simulink model "GT_cruise"  (R2024a)
settings: Solver=ode4  StartTime=0.0  StopTime=10  FixedStep=1/1600  RelTol=1e-3
undefined symbols (not defined in the file): wind_x, wind_y, wind_z
libraries: GT x1, aerolibasang x1
settings Model: Creator=igmso  LastModifiedBy=igmso
settings DataIOCC: ExternalInput=[t,u]  InitialState=getstatestruct(op_trim3)  SaveFormat=StructureWithTime

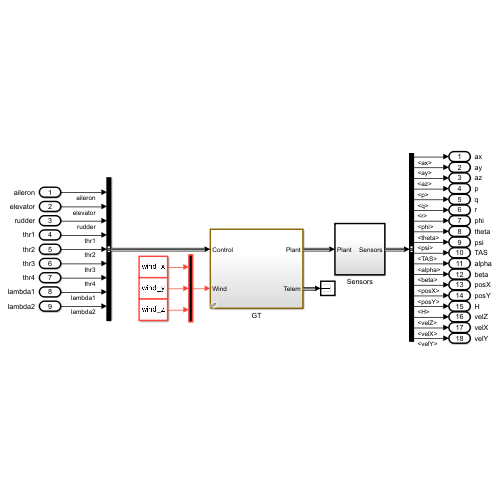
[thumbnail: Simulink's stored preview of the top-level diagram]
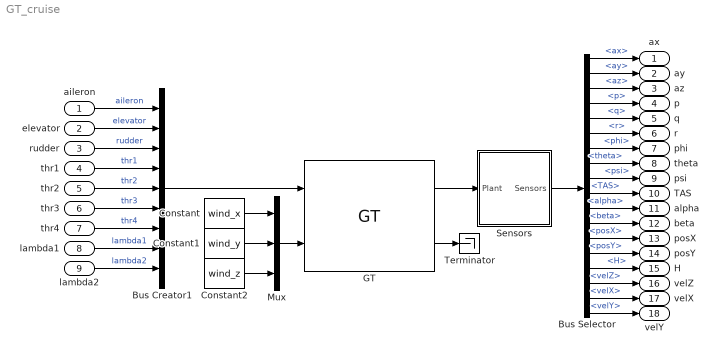
== system GT_cruise ==
  aileron : Inport
  elevator : Inport  Port=2
  rudder : Inport  Port=3
  thr1 : Inport  Port=4
  thr2 : Inport  Port=5
  thr3 : Inport  Port=6
  thr4 : Inport  Port=7
  lambda1 : Inport  Port=8
  lambda2 : Inport  Port=9
  Bus Creator1 : BusCreator  Inputs=9
  Bus Selector : BusSelector  OutputSignals=ax,ay,az,p,q,r,phi,theta,psi,TAS,alpha,beta,posX,posY,H,velZ,velX,velY
  Constant : Constant  Value=wind_x  SampleTime=-1
  Constant1 : Constant  Value=wind_y  SampleTime=-1
  Constant2 : Constant  Value=wind_z  SampleTime=-1
  GT : GT/GT  SystemSampleTime=-1  VariantActivationTime=update diagram  AllowFlexibleInterface=on  Latency=0  AutoFrameSizeCalculation=off
  Mux : Mux  Inputs=3
  Sensors : Subsystem
  Terminator : Terminator
  ax : Outport
  ay : Outport  Port=2
  az : Outport  Port=3
  p : Outport  Port=4
  q : Outport  Port=5
  r : Outport  Port=6
  phi : Outport  Port=7
  theta : Outport  Port=8
  psi : Outport  Port=9
  TAS : Outport  Port=10
  alpha : Outport  Port=11
  beta : Outport  Port=12
  posX : Outport  Port=13
  posY : Outport  Port=14
  H : Outport  Port=15
  velZ : Outport  Port=16
  velX : Outport  Port=17
  velY : Outport  Port=18
  wires:
  Bus Creator1/1 -> GT/1
  lambda2/1 -> Bus Creator1/9  "lambda2"
  lambda1/1 -> Bus Creator1/8  "lambda1"
  thr2/1 -> Bus Creator1/5  "thr2"
  thr3/1 -> Bus Creator1/6  "thr3"
  rudder/1 -> Bus Creator1/3  "rudder"
  thr1/1 -> Bus Creator1/4  "thr1"
  elevator/1 -> Bus Creator1/2  "elevator"
  aileron/1 -> Bus Creator1/1  "aileron"
  thr4/1 -> Bus Creator1/7  "thr4"
  Mux/1 -> GT/2
  Constant/1 -> Mux/1
  Constant1/1 -> Mux/2
  Constant2/1 -> Mux/3
  GT/2 -> Terminator/1
  GT/1 -> Sensors/1(Plant)
  Sensors/1(Sensors) -> Bus Selector/1
  Bus Selector/18 -> velY/1  "<velY>"
  Bus Selector/8 -> theta/1  "<theta>"
  Bus Selector/10 -> TAS/1  "<TAS>"
  Bus Selector/6 -> r/1  "<r>"
  Bus Selector/1 -> ax/1  "<ax>"
  Bus Selector/5 -> q/1  "<q>"
  Bus Selector/7 -> phi/1  "<phi>"
  Bus Selector/3 -> az/1  "<az>"
  Bus Selector/4 -> p/1  "<p>"
  Bus Selector/9 -> psi/1  "<psi>"
  Bus Selector/15 -> H/1  "<H>"
  Bus Selector/17 -> velX/1  "<velX>"
  Bus Selector/12 -> beta/1  "<beta>"
  Bus Selector/11 -> alpha/1  "<alpha>"
  Bus Selector/16 -> velZ/1  "<velZ>"
  Bus Selector/2 -> ay/1  "<ay>"
  Bus Selector/14 -> posY/1  "<posY>"
  Bus Selector/13 -> posX/1  "<posX>"

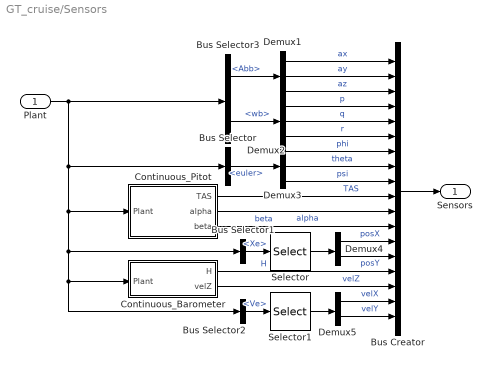
== system GT_cruise/Sensors ==
  Plant : Inport
  Bus Selector : BusSelector  OutputSignals=euler
  Bus Selector1 : BusSelector  OutputSignals=Xe
  Bus Selector2 : BusSelector  OutputSignals=Ve
  Bus Selector3 : BusSelector  OutputSignals=Abb,wb
  Bus Creator : BusCreator  Inputs=18
  Continuous_Barometer : Subsystem
  Continuous_Pitot : Subsystem
  Demux1 : Demux  Outputs=3
  Demux2 : Demux  Outputs=3
  Demux3 : Demux  Outputs=3
  Demux4 : Demux  Outputs=2
  Demux5 : Demux  Outputs=2
  Selector : Selector  InputPortWidth=3  IndexOptions=Index vector (dialog)  Indices=[1 2]  OutputSizes=1
  Selector1 : Selector  InputPortWidth=3  IndexOptions=Index vector (dialog)  Indices=[1 2]  OutputSizes=1
  Sensors : Outport
  wires:
  Continuous_Barometer/1(H) -> Bus Creator/15  "H"
  Continuous_Pitot/1(TAS) -> Bus Creator/10  "TAS"
  Continuous_Pitot/2(alpha) -> Bus Creator/11  "alpha"
  Continuous_Pitot/3(beta) -> Bus Creator/12  "beta"
  Demux1/3 -> Bus Creator/3  "az"
  Demux1/2 -> Bus Creator/2  "ay"
  Demux1/1 -> Bus Creator/1  "ax"
  Bus Selector3/1 -> Demux1/1  "<Abb>"
  Bus Selector3/2 -> Demux2/1  "<wb>"
  Demux2/1 -> Bus Creator/4  "p"
  Demux2/2 -> Bus Creator/5  "q"
  Demux2/3 -> Bus Creator/6  "r"
  Continuous_Barometer/2(velZ) -> Bus Creator/16  "velZ"
  Bus Selector/1 -> Demux3/1  "<euler>"
  Demux3/1 -> Bus Creator/7  "phi"
  Demux3/2 -> Bus Creator/8  "theta"
  Demux3/3 -> Bus Creator/9  "psi"
  Bus Selector1/1 -> Selector/1  "<Xe>"
  Selector/1 -> Demux4/1
  Demux4/1 -> Bus Creator/13  "posX"
  Demux4/2 -> Bus Creator/14  "posY"
  Bus Creator/1 -> Sensors/1
  Selector1/1 -> Demux5/1
  Bus Selector2/1 -> Selector1/1  "<Ve>"
  Plant/1 -> Bus Selector2/1, Continuous_Barometer/1(Plant), Bus Selector1/1, Continuous_Pitot/1(Plant), Bus Selector/1, Bus Selector3/1
  Demux5/1 -> Bus Creator/17  "velX"
  Demux5/2 -> Bus Creator/18  "velY"

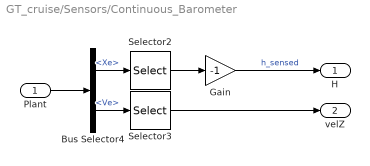
== system GT_cruise/Sensors/Continuous_Barometer ==
  Plant : Inport
  Bus Selector4 : BusSelector  OutputSignals=Xe,Ve
  Gain : Gain  Gain=-1
  Selector2 : Selector  InputPortWidth=3  IndexOptions=Index vector (dialog)  Indices=3  OutputSizes=1
  Selector3 : Selector  InputPortWidth=3  IndexOptions=Index vector (dialog)  Indices=3  OutputSizes=1
  H : Outport
  velZ : Outport  Port=2
  wires:
  Bus Selector4/1 -> Selector2/1  "<Xe>"
  Selector3/1 -> velZ/1
  Selector2/1 -> Gain/1
  Bus Selector4/2 -> Selector3/1  "<Ve>"
  Gain/1 -> H/1  "h_sensed"
  Plant/1 -> Bus Selector4/1

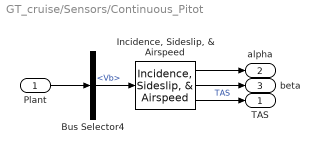
== system GT_cruise/Sensors/Continuous_Pitot ==
  Plant : Inport
  Bus Selector4 : BusSelector  OutputSignals=Vb
  "Incidence, Sideslip, & Airspeed" : aerolibasang/Incidence, Sideslip, & Airspeed
  TAS : Outport
  alpha : Outport  Port=2
  beta : Outport  Port=3
  wires:
  Bus Selector4/1 -> "Incidence, Sideslip, & Airspeed"/1  "<Vb>"
  "Incidence, Sideslip, & Airspeed"/1 -> alpha/1
  Plant/1 -> Bus Selector4/1
  "Incidence, Sideslip, & Airspeed"/3 -> TAS/1  "TAS"
  "Incidence, Sideslip, & Airspeed"/2 -> beta/1
